simulink model "gm_fixedpoint"  (R2022a)
settings: Solver=VariableStepAuto  StartTime=0.0  StopTime=1000.0  RelTol=1e-3
settings Model: Creator=Natriya  LastModifiedBy=Natriya
settings OptimizationCC: BlockReduction=off  ConditionallyExecuteInputs=off
settings DebuggingCC: InheritedTsInSrcMsg=none

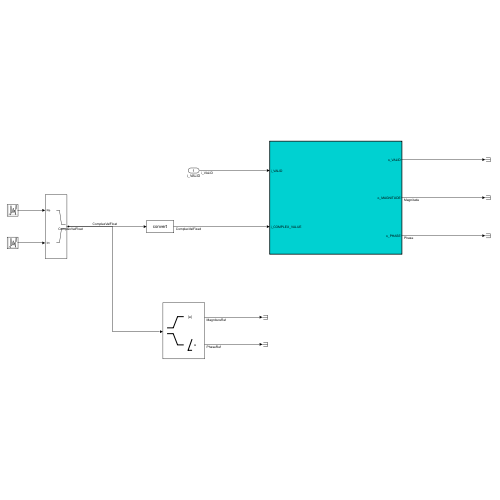
[thumbnail: Simulink's stored preview of the top-level diagram]
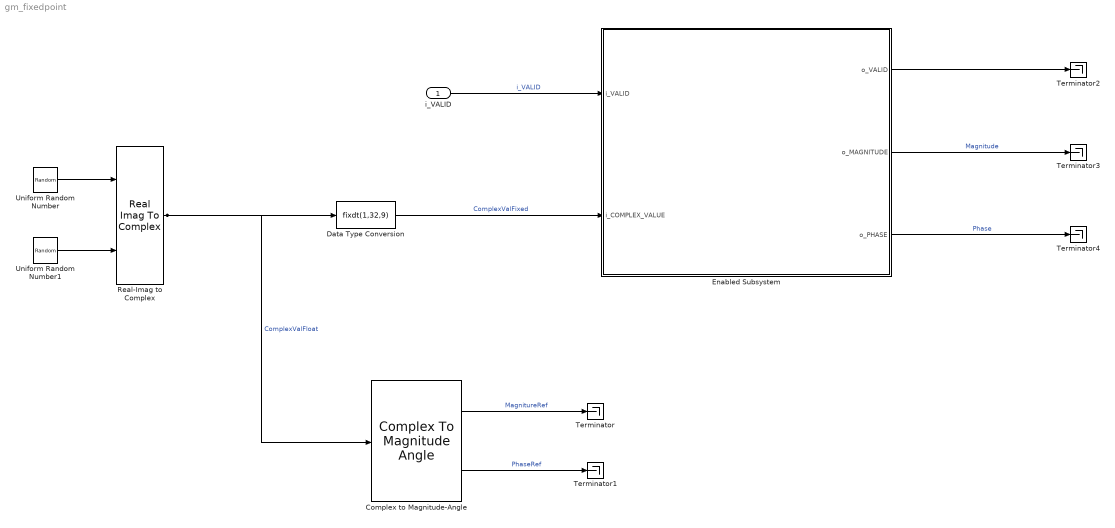
== system gm_fixedpoint ==
  i_VALID : Inport
  Complex to Magnitude-Angle : ComplexToMagnitudeAngle
  Data Type Conversion : DataTypeConversion  OutDataTypeStr=fixdt(1,32,9)  RndMeth=Round  SaturateOnIntegerOverflow=off
  Enabled Subsystem : Subsystem  TreatAsAtomicUnit=on
  Real-Imag to Complex : RealImagToComplex
  Terminator{,1..4} (5 alike) : Terminator
  Uniform Random Number : UniformRandomNumber  Minimum=-2^(23-1)  Maximum=2^(23-1)-1/2^9  Seed=23  SampleTime=1
  Uniform Random Number1 : UniformRandomNumber  Minimum=-2^(23-1)  Maximum=2^(23-1)-1/2^9  Seed=24  SampleTime=1
  wires:
  Enabled Subsystem/1(o_VALID) -> Terminator2/1
  Enabled Subsystem/2(o_MAGNITUDE) -> Terminator3/1  "Magnitude"
  Enabled Subsystem/3(o_PHASE) -> Terminator4/1  "Phase"
  Complex to Magnitude-Angle/2 -> Terminator1/1  "PhaseRef"
  Complex to Magnitude-Angle/1 -> Terminator/1  "MagnitureRef"
  i_VALID/1 -> Enabled Subsystem/1(i_VALID)  "i_VALID"
  Data Type Conversion/1 -> Enabled Subsystem/2(i_COMPLEX_VALUE)  "ComplexValFixed"
  Real-Imag to Complex/1 -> Data Type Conversion/1, Complex to Magnitude-Angle/1  "ComplexValFloat"
  Uniform Random Number/1 -> Real-Imag to Complex/1
  Uniform Random Number1/1 -> Real-Imag to Complex/2

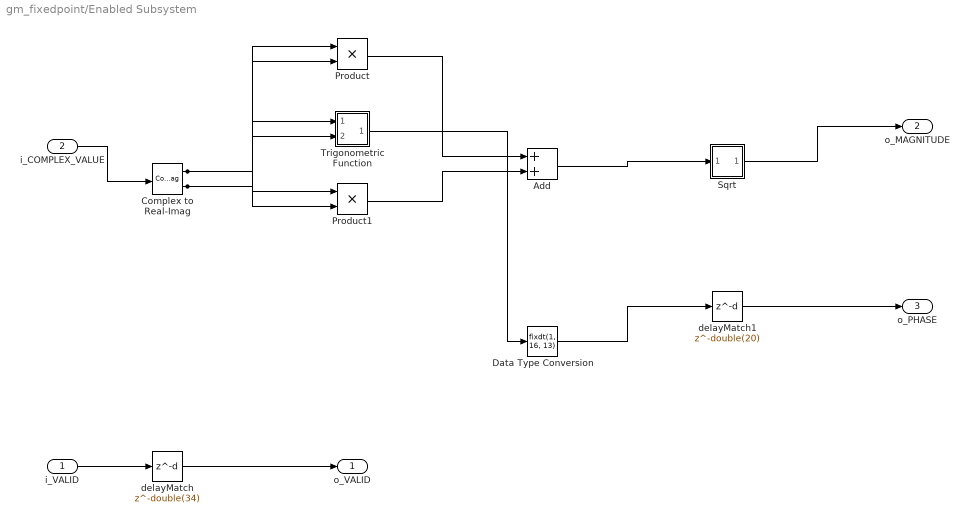
== system gm_fixedpoint/Enabled Subsystem ==
  i_VALID : Inport  OutDataTypeStr=double  PortDimensions=1  SampleTime=1
  i_COMPLEX_VALUE : Inport  Port=2  OutDataTypeStr=fixdt(1, 32, 9)  PortDimensions=1  SampleTime=1
      settings: SignalType=complex
  Add : Sum  AccumDataTypeStr=fixdt(1, 64, 18)  OutDataTypeStr=fixdt(1, 64, 18)  SampleTime=1
  Complex to Real-Imag : ComplexToRealImag  SampleTime=1
  Data Type Conversion : DataTypeConversion  OutDataTypeStr=fixdt(1, 16, 13)  SampleTime=1  SaturateOnIntegerOverflow=off  RndMeth=Floor
  Product : Product  Inputs=**  OutDataTypeStr=fixdt(1, 64, 18)  SampleTime=1
  Product1 : Product  Inputs=**  OutDataTypeStr=fixdt(1, 64, 18)  SampleTime=1
  Sqrt : Subsystem
  Trigonometric Function : Subsystem
  delayMatch : Delay  DelayLength=double(34)  InitialCondition=0  SampleTime=1
  delayMatch1 : Delay  DelayLength=double(20)  InitialCondition=0  SampleTime=1
  o_VALID : Outport  SampleTime=1
  o_MAGNITUDE : Outport  Port=2  SampleTime=1  VectorParamsAs1DForOutWhenUnconnected=off
  o_PHASE : Outport  Port=3  SampleTime=1  VectorParamsAs1DForOutWhenUnconnected=off
  wires:
  delayMatch/1 -> o_VALID/1
  i_COMPLEX_VALUE/1 -> Complex to Real-Imag/1
  Add/1 -> Sqrt/1(In1)
  Complex to Real-Imag/1 -> Product/2, Product/1, Trigonometric Function/2(In2)
  Complex to Real-Imag/2 -> Product1/2, Product1/1, Trigonometric Function/1(In1)
  delayMatch1/1 -> o_PHASE/1
  Product/1 -> Add/1
  Product1/1 -> Add/2
  Sqrt/1(Out1) -> o_MAGNITUDE/1
  Trigonometric Function/1(Out1) -> Data Type Conversion/1
  i_VALID/1 -> delayMatch/1
  Data Type Conversion/1 -> delayMatch1/1

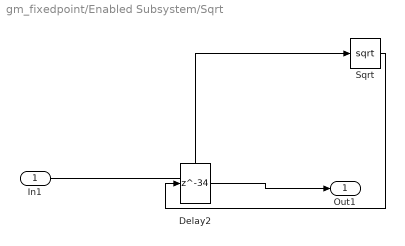
== system gm_fixedpoint/Enabled Subsystem/Sqrt ==
  In1 : Inport
  Delay2 : Delay  DelayLength=34
  Sqrt : Sqrt  OutDataTypeStr=fixdt(1,33,9)
  Out1 : Outport
  wires:
  In1/1 -> Sqrt/1
  Sqrt/1 -> Delay2/1
  Delay2/1 -> Out1/1

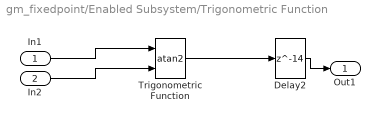
== system gm_fixedpoint/Enabled Subsystem/Trigonometric Function ==
  In1 : Inport
  In2 : Inport  Port=2
  Delay2 : Delay  DelayLength=14
  Trigonometric Function : Trigonometry  Operator=atan2  ApproximationMethod=CORDIC
  Out1 : Outport
  wires:
  In1/1 -> Trigonometric Function/1
  In2/1 -> Trigonometric Function/2
  Trigonometric Function/1 -> Delay2/1
  Delay2/1 -> Out1/1
